simulink library "vmc"  (R2021b)
settings: Solver=VariableStepAuto  StartTime=0.0  StopTime=10.0  RelTol=1e-3
undefined symbols (not defined in the file or in its folder): AVMC_ACCDeltaTqIGain_X_kph, AVMC_ACCDeltaTqIGain_Y_mps2, AVMC_ACCDeltaTqPGain_X_kph, AVMC_ACCDeltaTqPGain_Y_kph, AVMC_ACCLongSteadyCtrl_X_kph, AVMC_AggressJerkPCT4AT_X_kph, AVMC_AggressJerkPCT_X_kph, AVMC_AggressLimitPCT4AT_X_kph, AVMC_AggressLimitPCT_X_kph, AVMC_CCLongSteadyCtrl_X_kph, AVMC_DISCDeltaTqIGain_X_kph, AVMC_DISCDeltaTqIGain_Y_mps2, AVMC_DISCDeltaTqPGain_X_kph, AVMC_DISCDeltaTqPGain_Y_kph, AVMC_DISCTrunAccJerk_X_s, AVMC_DISCTrunAccLimit_X_s, AVMC_ESCRegenOut_X_kph, AVMC_ESCRegenOut_Y_Deg, AVMC_ESCRegenOutEnSpd_X_Deg, AVMC_ISOAccLimit_X_mps, AVMC_ISODecLimit_X_mps, AVMC_ISOJerk_X_mps, AVMC_LatESCRegenOut_X_kph, AVMC_LatESCRegenOut_Y_Deg, AVMC_LongAccDeadZone_X_kph, AVMC_LongAccFiltTsforP2_X_Gps, AVMC_MCPresBaseTq_X_bar, AVMC_MSALongSteadyCtrl_X_kph, AVMC_MSAPedalOvrd2_X_kph, AVMC_MSAPedalOvrd_X_kph, AVMC_MSASpdBand_X_kph, AVMC_MSATqDownEndTq_X_kph, AVMC_MSATqDownTime_X_kph, AVMC_RDCDetectTime_X_kph, AVMC_RDCDetectTime_Y_pct, AVMC_RDCEnSlideRate_X_Deg, AVMC_RearWhlTqRatio_X_Nm, AVMC_RearWhlTqRatio_Y_gps, AVMC_RearWhlTqSlipGain_X_rat, AVMC_RearWhlTqSlipGain_Y_kph, AVMC_SoftJerkPCT_X_kph, AVMC_SoftLimitPCT_X_kph, AVMC_StESCYaw_X_kph, AVMC_StESCYaw_Y_Deg, AVMC_StESCYawCom_X_kph, AVMC_StESCYawCom_Y_Gps, AVMC_TMSpdBaseTq_X_rpm, AVMC_VehHoldBDecMap_X_kph, AVMC_VehHoldDecCtrlTime_X_kph, AVMC_VehHoldMCPPass_X_deg, C_TASK_10MS_S, C_TASK_5MS_S, DEG2RAD, Discrete, ENUM_ACCAVAIL_AVAILABLE, ENUM_ACCCTRLALLOW_ALLOW, ENUM_ADASACCSTA_ACTIVE, ENUM_ADASACCSTA_OVERRIDE, ENUM_ADASACCSTA_SHUTOFF, ENUM_ADASAEBREQ_NOREQUEST ... (+361)
libraries: hcu_lib x63, simulink x60, simulink_extras x3, ctrlSharedLib x3, $bdroot x2
(part 5 of 15)

== system vmc/VMC/VMC/SpeedCalculation ==
  VINP_MeterIndVehSpeed_kph : Inport
  VINP_Distanceunit_flg : Inport  Port=2
  VINP_VehSpeed_kph : Inport  Port=3
  function : TriggerPort  TriggerType=function-call  VariantControl=(inherit)
  Add8 : Sum
  Cast To Single1 : DataTypeConversion  OutDataTypeStr=uint8
  Cast To Single{2..3,6..7,10..12} (7 alike) : DataTypeConversion  OutDataTypeStr=single
  Cast To Single13 : DataTypeConversion  OutDataTypeStr=uint8
  Constant1 : Constant  Value=KVMC_MeterSpdRoundSW_flg
  Constant11 : Constant  Value=KPH2MPH
  Constant19 : Constant  Value=KPH2MPH
  Constant2 : Constant  Value=KVMC_MeterSpdRoundSW_flg
  Constant22 : Constant  Value=C_TASK_10MS_S
  Constant23 : Constant  Value=KVMC_MeterSpdBWFilter_raw32
  Constant4 : Constant  Value=ONE_INT
  Constant5 : Constant  Value=KVMC_MeterSpdRollAveLevel_enum
  Constant7 : Constant  Value=ZERO_FLOAT
  Divide : Product  Inputs=**
  Divide2 : Product  Inputs=**
  FirstOrderFilter6 : hcu_lib/Basic_Blocks/FirstOrderFilter
  RollingAverage : Stateflow chart  TreatAsAtomicUnit=on
  Round : Rounding
  Round1 : Rounding  Operator=round
  Round2 : Rounding
  Round3 : Rounding  Operator=round
  u2 > 0 (1) : Switch  Criteria=u2 > Threshold
  u2 > 0 (1)1 : Switch  Criteria=u2 > Threshold
  u2 > 0 (1)2 : Switch  Criteria=u2 > Threshold
  VVMC_MeterIndSpeed_raw32 : Outport
  VVMC_VehicleSpeed_mph : Outport  Port=2
  VVMC_VehicleSpeed_kph : Outport  Port=3
  VVMC_MeterIndSpeedForCalcu_kph : Outport  Port=4
  wires:
  u2 > 0 (1)/1 -> Cast To Single6/1
  VINP_Distanceunit_flg/1 -> [VINP_Distanceunit_flg]
  [VINP_Distanceunit_flg] -> u2 > 0 (1)/2
  FirstOrderFilter6/1 -> [VVMC_MeterSpdRollAve_kph]  "VVMC_MeterSpdRollAve_kph"
  [VVMC_MeterIndSpeed_raw32] -> VVMC_MeterIndSpeed_raw32/1
  Constant19/1 -> Divide/2
  u2 > 0 (1)2/1 -> [VVMC_MeterIndSpeedForCalcu_kph]  "VVMC_MeterIndSpeedForCalcu_kph"
  [VVMC_VehicleSpeed_kph] -> VVMC_VehicleSpeed_kph/1
  Cast To Single6/1 -> Round1/1, Round/1
  Constant11/1 -> Divide2/2
  Cast To Single2/1 -> Divide2/1
  [VVMC_MeterIndSpeedForCalcu_kph] -> VVMC_MeterIndSpeedForCalcu_kph/1
  u2 > 0 (1)1/1 -> [VVMC_MeterIndSpeed_raw32]  "VVMC_MeterIndSpeed_raw32"
  VINP_VehSpeed_kph/1 -> [VINP_VehSpeed_kph]
  Divide/1 -> u2 > 0 (1)/1
  [VVMC_MeterSpdRollAve_kph] -> Cast To Single7/1, u2 > 0 (1)/3, Round2/1, Round3/1  "VVMC_MeterSpdRollAve_kph"
  [VINP_VehSpeed_kph] -> Cast To Single10/1, Cast To Single2/1
  Cast To Single7/1 -> Divide/1
  VINP_MeterIndVehSpeed_kph/1 -> [VINP_MeterIndVehSpeed_kph]
  Divide2/1 -> [VVMC_VehicleSpeed_mph]  "VVMC_VehicleSpeed_mph"
  Cast To Single10/1 -> [VVMC_VehicleSpeed_kph]  "VVMC_VehicleSpeed_kph"
  [VVMC_VehicleSpeed_mph] -> VVMC_VehicleSpeed_mph/1
  Constant22/1 -> Add8/1, FirstOrderFilter6/2
  Add8/1 -> FirstOrderFilter6/3
  Constant23/1 -> Add8/2
  Cast To Single3/1 -> FirstOrderFilter6/1
  Constant1/1 -> u2 > 0 (1)1/2
  Round/1 -> u2 > 0 (1)1/3
  Round1/1 -> u2 > 0 (1)1/1
  Round2/1 -> u2 > 0 (1)2/3
  Constant2/1 -> u2 > 0 (1)2/2
  Round3/1 -> u2 > 0 (1)2/1
  RollingAverage/1(VVMC_MeterSpdRollAve_kph) -> Cast To Single3/1
  Constant5/1 -> Cast To Single1/1
  [VINP_MeterIndVehSpeed_kph] -> Cast To Single12/1
  Constant4/1 -> Cast To Single13/1
  Constant7/1 -> Cast To Single11/1
  Cast To Single12/1 -> RollingAverage/4(VINP_MeterIndVehSpeed_kph)
  Cast To Single13/1 -> RollingAverage/3(ONE_INT)
  Cast To Single11/1 -> RollingAverage/2(ZERO_FLOAT)
  Cast To Single1/1 -> RollingAverage/1(KVMC_MeterSpdRollAveLevel_enum)

== system vmc/VMC/VMC/Triggered Subsystem ==
  In1 : Inport
  Trigger : TriggerPort  VariantControl=(inherit)
  Out1 : Outport
  wires:
  In1/1 -> Out1/1

== system vmc/VMC/VMC/Triggered Subsystem1 ==
  In1 : Inport
  Trigger : TriggerPort  VariantControl=(inherit)
  Out1 : Outport
  wires:
  In1/1 -> Out1/1

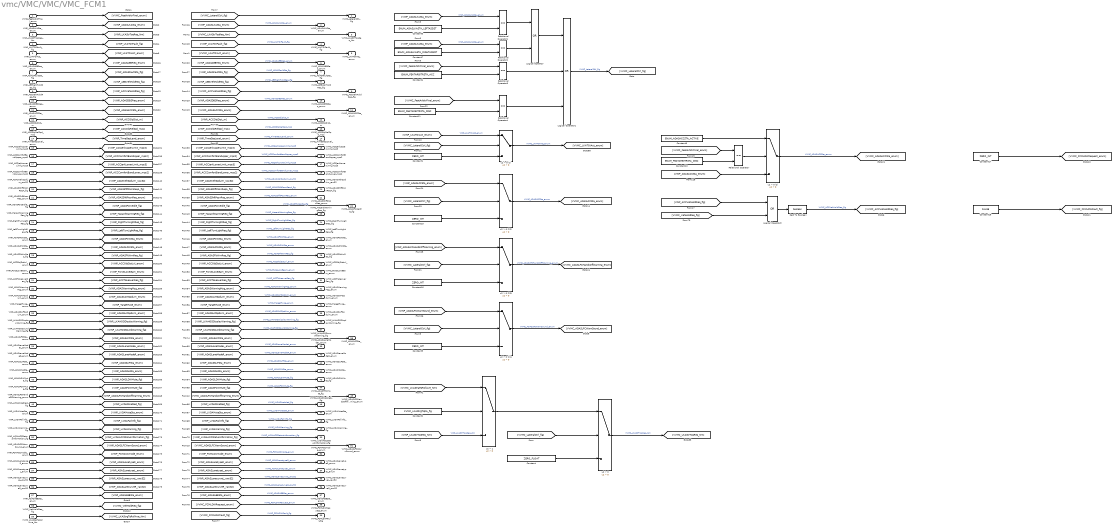
== system vmc/VMC/VMC/VMC_FCM1 ==
  VVMC_FeatArbitrFinal_enum : Inport
  VINP_ADASLKASta_enum : Inport  Port=2
  VINP_LKAStrToqReq_Nm : Inport  Port=3
  VINP_LKATOIFault_flg : Inport  Port=4
  VINP_LKATOIAct_enum : Inport  Port=5
  VINP_ADASAEBReq_enum : Inport  Port=6
  VINP_ADASFaultSta_flg : Inport  Port=7
  VINP_AEBVehHoldReq_flg : Inport  Port=8
  VINP_ACCVehHoldReq_flg : Inport  Port=9
  VINP_ADASDBSReq_enum : Inport  Port=10
  VINP_ADASACCSta_enum : Inport  Port=11
  VINP_ACCObjDist_m : Inport  Port=12
  VINP_ACCObjRelSpd_mps : Inport  Port=13
  VINP_TimeGapLevel_enum : Inport  Port=14
  VINP_ACCJerkUpperLimit_mps3 : Inport  Port=15
  VINP_ACCComfortBandUpper_mps2 : Inport  Port=16
  VINP_ACCJerkLowerLimit_mps3 : Inport  Port=17
  VINP_ACCComfortBandLower_mps2 : Inport  Port=18
  VINP_ADASVehSpdLim_raw32 : Inport  Port=19
  VINP_ADASShftPosnReqA_flg : Inport  Port=20
  VINP_ADASShftPosnReq_enum : Inport  Port=21
  VINP_ADASForceIdle_flg : Inport  Port=22
  VINP_HazardWarningReq_flg : Inport  Port=23
  VINP_RightTurnLightReq_flg : Inport  Port=24
  VINP_LeftTurnLightReq_flg : Inport  Port=25
  VINP_ADASFCWSta_enum : Inport  Port=26
  VINP_ADASLDWSta_enum : Inport  Port=27
  VINP_ADASFltWrnReq_flg : Inport  Port=28
  VINP_ACCObjDstLvl_enum : Inport  Port=29
  VINP_ForceLowBeam_enum : Inport  Port=30
  VINP_ACCTakeoverReq_flg : Inport  Port=31
  VINP_ADASWarningMsg_enum : Inport  Port=32
  VINP_ADASCAMSpdLim_enum : Inport  Port=33
  VINP_TargetType_enum : Inport  Port=34
  VINP_ADASSLIFSpdLim_enum : Inport  Port=35
  VINP_LKAHODDisplayWarning_flg : Inport  Port=36
  VINP_LKAHODSoundWarning_flg : Inport  Port=37
  VINP_ADASLFCSta_enum : Inport  Port=38
  VINP_ADASLaneModeL_enum : Inport  Port=39
  VINP_ADASLaneModeR_enum : Inport  Port=40
  VINP_ADASSLIFSta_enum : Inport  Port=41
  VINP_ADASISASta_enum : Inport  Port=42
  VINP_ADASLDWMute_flg : Inport  Port=43
  VINP_ADASFCWMute_flg : Inport  Port=44
  VINP_ADASLFCHandsOffWarning_enum : Inport  Port=45
  VINP_LVDADisabled_flg : Inport  Port=46
  VINP_LVDAMuteSta_enum : Inport  Port=47
  VINP_LVDAFailinfo_flg : Inport  Port=48
  VINP_LVDAWarning_flg : Inport  Port=49
  VINP_LVDAACCStatusInformation_flg : Inport  Port=50
  VINP_ADASLFCWarnSound_enum : Inport  Port=51
  VINP_FCMACCmode_enum : Inport  Port=52
  VINP_ADASLanetypeR_enum : Inport  Port=53
  VINP_ADASLanetypeL_enum : Inport  Port=54
  VINP_ADASLanecurveL_raw32 : Inport  Port=55
  VINP_ADASLanecurveR_raw32 : Inport  Port=56
  VINP_ADASAEBSta_enum : Inport  Port=57
  VVMC_VehHoldReq_flg : Inport  Port=58
  VVMC_LKAStrgTqRollAve_Nm : Inport  Port=59
  Cast To Boolean : DataTypeConversion  OutDataTypeStr=boolean
  Constant : Constant  Value=ZERO_FLOAT
  Constant{1,3,15..17} (5 alike) : Constant  Value=ZERO_INT
  Constant10 : Constant  Value=ENUM_FEATARBITRSTA_DISC
  Constant11 : Constant  Value=ENUM_FEATARBITRSTA_DISC
  Constant18 : Constant  Value=FALSE
  Constant2 : Constant  Value=KVMC_LKAStrgTqRA_flg
  Constant4 : Constant  Value=ENUM_FEATARBITRSTA_ACC
  Constant6 : Constant  Value=ENUM_ADASLKASTA_LEFTASSIST
  Constant7 : Constant  Value=ENUM_ADASLKASTA_RIGHTASSIST
  Constant9 : Constant  Value=ENUM_ADASACCSTA_ACTIVE
  Logical Operator : Logic  Operator=OR  AllPortsSameDT=off  OutDataTypeStr=boolean
  Logical Operator1 : Logic  Operator=OR  Inputs=3  AllPortsSameDT=off  OutDataTypeStr=boolean
  Logical Operator2 : Logic  Operator=OR  AllPortsSameDT=off  OutDataTypeStr=boolean
  Relational Operator{,1..4} (5 alike) : RelationalOperator  Operator===  OutDataTypeStr=boolean  RndMeth=Simplest
  u2 > 0 : Switch  Criteria=u2 > Threshold
  u2 > 0 (1) : Switch  Criteria=u2 > Threshold
  u2 > 0 (2){,2..4} (4 alike) : Switch  Criteria=u2 > Threshold
  u2 > 1 : Switch  Criteria=u2 > Threshold
  VVMC_LateralCtrl_flg : Outport
  VVMC_ADASLKASta_enum : Outport  Port=2
  VVMC_LKAStrToqReq_Nm : Outport  Port=3
  VVMC_LKATOIFault_flg : Outport  Port=4
  VVMC_LKATOIAct_enum : Outport  Port=5
  VVMC_ADASAEBReq_enum : Outport  Port=6
  VVMC_ADASFaultSta_flg : Outport  Port=7
  VVMC_AEBVehHoldReq_flg : Outport  Port=8
  VVMC_ACCVehHoldReq_flg : Outport  Port=9
  VVMC_ADASDBSReq_enum : Outport  Port=10
  VVMC_ADASACCSta_enum : Outport  Port=11
  VVMC_ACCObjDist_m : Outport  Port=12
  VVMC_ACCObjRelSpd_mps : Outport  Port=13
  VVMC_TimeGapLevel_enum : Outport  Port=14
  VVMC_ACCJerkUpperLimit_mps3 : Outport  Port=15
  VVMC_ACCComfortBandUpper_mps2 : Outport  Port=16
  VVMC_ACCJerkLowerLimit_mps3 : Outport  Port=17
  VVMC_ACCComfortBandLower_mps2 : Outport  Port=18
  VVMC_ADASVehSpdLim_raw32 : Outport  Port=19
  VVMC_ADASShftPosnReqA_flg : Outport  Port=20
  VVMC_ADASShftPosnReq_enum : Outport  Port=21
  VVMC_ADASForceIdle_flg : Outport  Port=22
  VVMC_HazardWarningReq_flg : Outport  Port=23
  VVMC_RightTurnLightReq_flg : Outport  Port=24
  VVMC_LeftTurnLightReq_flg : Outport  Port=25
  VVMC_ADASFCWSta_enum : Outport  Port=26
  VVMC_ADASLDWSta_enum : Outport  Port=27
  VVMC_ADASFltWrnReq_flg : Outport  Port=28
  VVMC_ACCObjDstLvl_enum : Outport  Port=29
  VVMC_ForceLowBeam_enum : Outport  Port=30
  VVMC_ACCTakeoverReq_flg : Outport  Port=31
  VVMC_ADASWarningMsg_enum : Outport  Port=32
  VVMC_ADASCAMSpdLim_enum : Outport  Port=33
  VVMC_TargetType_enum : Outport  Port=34
  VVMC_ADASSLIFSpdLim_enum : Outport  Port=35
  VVMC_LKAHODDisplayWarning_flg : Outport  Port=36
  VVMC_LKAHODSoundWarning_flg : Outport  Port=37
  VVMC_ADASLFCSta_enum : Outport  Port=38
  VVMC_ADASLaneModeL_enum : Outport  Port=39
  VVMC_ADASLaneModeR_enum : Outport  Port=40
  VVMC_ADASSLIFSta_enum : Outport  Port=41
  VVMC_ADASISASta_enum : Outport  Port=42
  VVMC_ADASLDWMute_flg : Outport  Port=43
  VVMC_ADASFCWMute_flg : Outport  Port=44
  VVMC_ADASLFCHandsOffWarning_enum : Outport  Port=45
  VVMC_LVDADisabled_flg : Outport  Port=46
  VVMC_LVDAMuteSta_enum : Outport  Port=47
  VVMC_LVDAFailinfo_flg : Outport  Port=48
  VVMC_LVDAWarning_flg : Outport  Port=49
  VVMC_LVDAACCStatusInformation_flg : Outport  Port=50
  VVMC_ADASLFCWarnSound_enum : Outport  Port=51
  VVMC_FCMACCmode_enum : Outport  Port=52
  VVMC_ADASLanetypeR_enum : Outport  Port=53
  VVMC_ADASLanetypeL_enum : Outport  Port=54
  VVMC_ADASLanecurveL_raw32 : Outport  Port=55
  VVMC_ADASLanecurveR_raw32 : Outport  Port=56
  VVMC_ADASAEBSta_enum : Outport  Port=57
  VVMC_FCMLDWRequest_enum : Outport  Port=58
  VVMC_FCMLDWFault_flg : Outport  Port=59
  wires:
  [VVMC_LateralCtrl_flg] -> VVMC_LateralCtrl_flg/1
  u2 > 0 (1)/1 -> [VVMC_LKATOIAct_enum]  "VVMC_LKATOIAct_enum"
  Constant1/1 -> u2 > 0 (1)/3
  [VVMC_LateralCtrl_flg] -> u2 > 0 (1)/2
  u2 > 0/1 -> [VVMC_LKAStrToqReq_Nm]  "VVMC_LKAStrToqReq_Nm"
  Constant/1 -> u2 > 0/3
  [VVMC_LateralCtrl_flg] -> u2 > 0/2
  Logical Operator1/1 -> [VVMC_LateralCtrl_flg]  "VVMC_LateralCtrl_flg"
  Relational Operator3/1 -> Logical Operator1/2
  Logical Operator/1 -> Logical Operator1/1
  Relational Operator2/1 -> Logical Operator/2
  Relational Operator1/1 -> Logical Operator/1
  [VINP_ADASLKASta_enum] -> Relational Operator2/1  "VINP_ADASLKASta_enum"
  [VINP_ADASLKASta_enum] -> Relational Operator1/1  "VINP_ADASLKASta_enum"
  [VVMC_FeatArbitrFinal_enum] -> Relational Operator3/1
  Constant4/1 -> Relational Operator3/2
  Constant6/1 -> Relational Operator1/2
  Constant7/1 -> Relational Operator2/2
  u2 > 1/1 -> u2 > 0/1
  [VINP_LKATOIAct_enum] -> u2 > 0 (1)/1  "VINP_LKATOIAct_enum"
  VINP_LKATOIAct_enum/1 -> [VINP_LKATOIAct_enum]
  VINP_LKATOIFault_flg/1 -> [VINP_LKATOIFault_flg]
  VINP_LKAStrToqReq_Nm/1 -> [VINP_LKAStrToqReq_Nm]
  VINP_ADASLKASta_enum/1 -> [VINP_ADASLKASta_enum]
  VVMC_FeatArbitrFinal_enum/1 -> [VVMC_FeatArbitrFinal_enum]
  VINP_ADASFaultSta_flg/1 -> [VINP_ADASFaultSta_flg]
  VINP_ADASAEBReq_enum/1 -> [VINP_ADASAEBReq_enum]
  VINP_AEBVehHoldReq_flg/1 -> [VINP_AEBVehHoldReq_flg]
  VINP_ADASDBSReq_enum/1 -> [VINP_ADASDBSReq_enum]
  VINP_ACCVehHoldReq_flg/1 -> [VINP_ACCVehHoldReq_flg]
  [VINP_ADASACCSta_enum] -> u2 > 0 (2)/3
  u2 > 0 (2)/1 -> [VVMC_ADASACCSta_enum]  "VVMC_ADASACCSta_enum"
  [VVMC_FeatArbitrFinal_enum] -> Relational Operator/1
  VINP_ADASACCSta_enum/1 -> [VINP_ADASACCSta_enum]
  Constant9/1 -> u2 > 0 (2)/1
  Constant10/1 -> Relational Operator/2
  Relational Operator/1 -> u2 > 0 (2)/2
  VINP_ACCJerkUpperLimit_mps3/1 -> [VINP_ACCJerkUpperLimit_mps3]
  VINP_ForceLowBeam_enum/1 -> [VINP_ForceLowBeam_enum]
  VINP_ADASLFCSta_enum/1 -> [VINP_ADASLFCSta_enum]
  VINP_ADASLanecurveR_raw32/1 -> [VINP_ADASLanecurveR_raw32]
  VINP_ADASLDWSta_enum/1 -> [VINP_ADASLDWSta_enum]
  VINP_ADASLaneModeR_enum/1 -> [VINP_ADASLaneModeR_enum]
  VINP_ACCComfortBandLower_mps2/1 -> [VINP_ACCComfortBandLower_mps2]
  VINP_ADASLanecurveL_raw32/1 -> [VINP_ADASLanecurveL_raw32]
  VINP_TargetType_enum/1 -> [VINP_TargetType_enum]
  VINP_ACCJerkLowerLimit_mps3/1 -> [VINP_ACCJerkLowerLimit_mps3]
  VINP_ADASShftPosnReq_enum/1 -> [VINP_ADASShftPosnReq_enum]
  VINP_ADASSLIFSta_enum/1 -> [VINP_ADASSLIFSta_enum]
  VINP_ADASShftPosnReqA_flg/1 -> [VINP_ADASShftPosnReqA_flg]
  VINP_LVDAMuteSta_enum/1 -> [VINP_LVDAMuteSta_enum]
  VINP_ACCComfortBandUpper_mps2/1 -> [VINP_ACCComfortBandUpper_mps2]
  VINP_FCMACCmode_enum/1 -> [VINP_FCMACCmode_enum]
  VINP_ADASCAMSpdLim_enum/1 -> [VINP_ADASCAMSpdLim_enum]
  VINP_LVDADisabled_flg/1 -> [VINP_LVDADisabled_flg]
  VINP_LKAHODDisplayWarning_flg/1 -> [VINP_LKAHODDisplayWarning_flg]
  VINP_ADASLDWMute_flg/1 -> [VINP_ADASLDWMute_flg]
  VINP_ADASFCWSta_enum/1 -> [VINP_ADASFCWSta_enum]
  VINP_LKAHODSoundWarning_flg/1 -> [VINP_LKAHODSoundWarning_flg]
  VINP_LeftTurnLightReq_flg/1 -> [VINP_LeftTurnLightReq_flg]
  VINP_ADASWarningMsg_enum/1 -> [VINP_ADASWarningMsg_enum]
  VINP_ADASFCWMute_flg/1 -> [VINP_ADASFCWMute_flg]
  VINP_ADASLanetypeL_enum/1 -> [VINP_ADASLanetypeL_enum]
  VINP_ADASFltWrnReq_flg/1 -> [VINP_ADASFltWrnReq_flg]
  VINP_RightTurnLightReq_flg/1 -> [VINP_RightTurnLightReq_flg]
  VINP_ACCTakeoverReq_flg/1 -> [VINP_ACCTakeoverReq_flg]
  VINP_ADASLFCWarnSound_enum/1 -> [VINP_ADASLFCWarnSound_enum]
  VINP_ACCObjDstLvl_enum/1 -> [VINP_ACCObjDstLvl_enum]
  VINP_LVDAFailinfo_flg/1 -> [VINP_LVDAFailinfo_flg]
  VINP_HazardWarningReq_flg/1 -> [VINP_HazardWarningReq_flg]
  VINP_ADASSLIFSpdLim_enum/1 -> [VINP_ADASSLIFSpdLim_enum]
  VINP_LVDAWarning_flg/1 -> [VINP_LVDAWarning_flg]
  VINP_ADASLFCHandsOffWarning_enum/1 -> [VINP_ADASLFCHandsOffWarning_enum]
  VINP_ADASLaneModeL_enum/1 -> [VINP_ADASLaneModeL_enum]
  VINP_ADASLanetypeR_enum/1 -> [VINP_ADASLanetypeR_enum]
  VINP_LVDAACCStatusInformation_flg/1 -> [VINP_LVDAACCStatusInformation_flg]
  VINP_ADASVehSpdLim_raw32/1 -> [VINP_ADASVehSpdLim_raw32]
  VINP_ADASForceIdle_flg/1 -> [VINP_ADASForceIdle_flg]
  VINP_ADASISASta_enum/1 -> [VINP_ADASISASta_enum]
  VINP_ACCObjRelSpd_mps/1 -> [VINP_ACCObjRelSpd_mps]
  VINP_ACCObjDist_m/1 -> [VINP_ACCObjDist_m]
  VINP_TimeGapLevel_enum/1 -> [VINP_TimeGapLevel_enum]
  [VINP_ACCVehHoldReq_flg] -> Logical Operator2/1
  Cast To Boolean/1 -> [VVMC_ACCVehHoldReq_flg]  "VVMC_ACCVehHoldReq_flg"
  Constant15/1 -> u2 > 0 (2)2/3
  u2 > 0 (2)2/1 -> [VVMC_ADASLFCSta_enum]  "VVMC_ADASLFCSta_enum"
  [VINP_ADASLFCSta_enum] -> u2 > 0 (2)2/1
  [VVMC_LateralCtrl_flg] -> u2 > 0 (2)2/2
  [VVMC_LateralCtrl_flg] -> u2 > 0 (2)3/2
  [VINP_ADASLFCHandsOffWarning_enum] -> u2 > 0 (2)3/1
  u2 > 0 (2)3/1 -> [VVMC_ADASLFCHandsOffWarning_enum]  "VVMC_ADASLFCHandsOffWarning_enum"
  Constant16/1 -> u2 > 0 (2)3/3
  Constant3/1 -> u2 > 0 (2)4/3
  u2 > 0 (2)4/1 -> [VVMC_ADASLFCWarnSound_enum]  "VVMC_ADASLFCWarnSound_enum"
  [VINP_ADASLFCWarnSound_enum] -> u2 > 0 (2)4/1
  [VVMC_LateralCtrl_flg] -> u2 > 0 (2)4/2
  [VINP_ADASLKASta_enum] -> VVMC_ADASLKASta_enum/1  "VVMC_ADASLKASta_enum"
  [VVMC_LKAStrToqReq_Nm] -> VVMC_LKAStrToqReq_Nm/1
  [VINP_LKATOIFault_flg] -> VVMC_LKATOIFault_flg/1  "VVMC_LKATOIFault_flg"
  [VVMC_LKATOIAct_enum] -> VVMC_LKATOIAct_enum/1
  [VINP_ADASAEBReq_enum] -> VVMC_ADASAEBReq_enum/1  "VVMC_ADASAEBReq_enum"
  [VINP_ADASFaultSta_flg] -> VVMC_ADASFaultSta_flg/1  "VVMC_ADASFaultSta_flg"
  [VINP_AEBVehHoldReq_flg] -> VVMC_AEBVehHoldReq_flg/1  "VVMC_AEBVehHoldReq_flg"
  [VVMC_ACCVehHoldReq_flg] -> VVMC_ACCVehHoldReq_flg/1
  [VINP_ADASDBSReq_enum] -> VVMC_ADASDBSReq_enum/1  "VVMC_ADASDBSReq_enum"
  [VVMC_ADASACCSta_enum] -> VVMC_ADASACCSta_enum/1
  [VINP_ACCObjDist_m] -> VVMC_ACCObjDist_m/1  "VVMC_ACCObjDist_m"
  [VINP_ACCObjRelSpd_mps] -> VVMC_ACCObjRelSpd_mps/1  "VVMC_ACCObjRelSpd_mps"
  [VINP_TimeGapLevel_enum] -> VVMC_TimeGapLevel_enum/1  "VVMC_TimeGapLevel_enum"
  [VINP_ACCJerkUpperLimit_mps3] -> VVMC_ACCJerkUpperLimit_mps3/1  "VVMC_ACCJerkUpperLimit_mps3"
  [VINP_ACCComfortBandUpper_mps2] -> VVMC_ACCComfortBandUpper_mps2/1  "VVMC_ACCComfortBandUpper_mps2"
  [VINP_ACCJerkLowerLimit_mps3] -> VVMC_ACCJerkLowerLimit_mps3/1  "VVMC_ACCJerkLowerLimit_mps3"
  [VINP_ACCComfortBandLower_mps2] -> VVMC_ACCComfortBandLower_mps2/1  "VVMC_ACCComfortBandLower_mps2"
  [VINP_ADASVehSpdLim_raw32] -> VVMC_ADASVehSpdLim_raw32/1  "VVMC_ADASVehSpdLim_raw32"
  [VINP_ADASShftPosnReqA_flg] -> VVMC_ADASShftPosnReqA_flg/1  "VVMC_ADASShftPosnReqA_flg"
  [VINP_ADASShftPosnReq_enum] -> VVMC_ADASShftPosnReq_enum/1  "VVMC_ADASShftPosnReq_enum"
  [VINP_ADASForceIdle_flg] -> VVMC_ADASForceIdle_flg/1  "VVMC_ADASForceIdle_flg"
  [VINP_HazardWarningReq_flg] -> VVMC_HazardWarningReq_flg/1  "VVMC_HazardWarningReq_flg"
  [VINP_RightTurnLightReq_flg] -> VVMC_RightTurnLightReq_flg/1  "VVMC_RightTurnLightReq_flg"
  [VINP_LeftTurnLightReq_flg] -> VVMC_LeftTurnLightReq_flg/1  "VVMC_LeftTurnLightReq_flg"
  [VINP_ADASFCWSta_enum] -> VVMC_ADASFCWSta_enum/1  "VVMC_ADASFCWSta_enum"
  [VINP_ADASLDWSta_enum] -> VVMC_ADASLDWSta_enum/1  "VVMC_ADASLDWSta_enum"
  [VINP_ADASFltWrnReq_flg] -> VVMC_ADASFltWrnReq_flg/1  "VVMC_ADASFltWrnReq_flg"
  [VINP_ACCObjDstLvl_enum] -> VVMC_ACCObjDstLvl_enum/1  "VVMC_ACCObjDstLvl_enum"
  [VINP_ForceLowBeam_enum] -> VVMC_ForceLowBeam_enum/1  "VVMC_ForceLowBeam_enum"
  [VINP_ACCTakeoverReq_flg] -> VVMC_ACCTakeoverReq_flg/1  "VVMC_ACCTakeoverReq_flg"
  [VINP_ADASWarningMsg_enum] -> VVMC_ADASWarningMsg_enum/1  "VVMC_ADASWarningMsg_enum"
  [VINP_ADASCAMSpdLim_enum] -> VVMC_ADASCAMSpdLim_enum/1  "VVMC_ADASCAMSpdLim_enum"
  [VINP_TargetType_enum] -> VVMC_TargetType_enum/1  "VVMC_TargetType_enum"
  [VINP_ADASSLIFSpdLim_enum] -> VVMC_ADASSLIFSpdLim_enum/1  "VVMC_ADASSLIFSpdLim_enum"
  [VINP_LKAHODDisplayWarning_flg] -> VVMC_LKAHODDisplayWarning_flg/1  "VVMC_LKAHODDisplayWarning_flg"
  [VINP_LKAHODSoundWarning_flg] -> VVMC_LKAHODSoundWarning_flg/1  "VVMC_LKAHODSoundWarning_flg"
  [VVMC_ADASLFCSta_enum] -> VVMC_ADASLFCSta_enum/1
  [VINP_ADASLaneModeL_enum] -> VVMC_ADASLaneModeL_enum/1  "VVMC_ADASLaneModeL_enum"
  [VINP_ADASLaneModeR_enum] -> VVMC_ADASLaneModeR_enum/1  "VVMC_ADASLaneModeR_enum"
  [VINP_ADASSLIFSta_enum] -> VVMC_ADASSLIFSta_enum/1  "VVMC_ADASSLIFSta_enum"
  [VINP_ADASISASta_enum] -> VVMC_ADASISASta_enum/1  "VVMC_ADASISASta_enum"
  [VINP_ADASLDWMute_flg] -> VVMC_ADASLDWMute_flg/1  "VVMC_ADASLDWMute_flg"
  [VINP_ADASFCWMute_flg] -> VVMC_ADASFCWMute_flg/1  "VVMC_ADASFCWMute_flg"
  [VVMC_ADASLFCHandsOffWarning_enum] -> VVMC_ADASLFCHandsOffWarning_enum/1
  [VINP_LVDADisabled_flg] -> VVMC_LVDADisabled_flg/1  "VVMC_LVDADisabled_flg"
  [VINP_LVDAMuteSta_enum] -> VVMC_LVDAMuteSta_enum/1  "VVMC_LVDAMuteSta_enum"
  [VINP_LVDAFailinfo_flg] -> VVMC_LVDAFailinfo_flg/1  "VVMC_LVDAFailinfo_flg"
  [VINP_LVDAWarning_flg] -> VVMC_LVDAWarning_flg/1  "VVMC_LVDAWarning_flg"
  [VINP_LVDAACCStatusInformation_flg] -> VVMC_LVDAACCStatusInformation_flg/1  "VVMC_LVDAACCStatusInformation_flg"
  [VVMC_ADASLFCWarnSound_enum] -> VVMC_ADASLFCWarnSound_enum/1
  [VINP_FCMACCmode_enum] -> VVMC_FCMACCmode_enum/1  "VVMC_FCMACCmode_enum"
  [VINP_ADASLanetypeR_enum] -> VVMC_ADASLanetypeR_enum/1  "VVMC_ADASLanetypeR_enum"
  [VINP_ADASLanetypeL_enum] -> VVMC_ADASLanetypeL_enum/1  "VVMC_ADASLanetypeL_enum"
  [VINP_ADASLanecurveL_raw32] -> VVMC_ADASLanecurveL_raw32/1  "VVMC_ADASLanecurveL_raw32"
  [VINP_ADASLanecurveR_raw32] -> VVMC_ADASLanecurveR_raw32/1  "VVMC_ADASLanecurveR_raw32"
  VINP_ADASAEBSta_enum/1 -> [VINP_ADASAEBSta_enum]
  [VINP_ADASAEBSta_enum] -> VVMC_ADASAEBSta_enum/1  "VVMC_ADASAEBSta_enum"
  Constant17/1 -> [VVMC_FCMLDWRequest_enum]
  Constant18/1 -> [VVMC_FCMLDWFault_flg]
  [VVMC_FCMLDWRequest_enum] -> VVMC_FCMLDWRequest_enum/1  "VVMC_FCMLDWRequest_enum"
  [VVMC_FCMLDWFault_flg] -> VVMC_FCMLDWFault_flg/1  "VVMC_FCMLDWFault_flg"
  VVMC_VehHoldReq_flg/1 -> [VVMC_VehHoldReq_flg]
  Logical Operator2/1 -> Cast To Boolean/1
  [VVMC_VehHoldReq_flg] -> Logical Operator2/2
  Constant11/1 -> Relational Operator4/2
  [VVMC_FeatArbitrFinal_enum] -> Relational Operator4/1
  Relational Operator4/1 -> Logical Operator1/3
  Constant2/1 -> u2 > 1/2
  [VINP_LKAStrToqReq_Nm] -> u2 > 1/3  "VINP_LKAStrToqReq_Nm"
  [VVMC_LKAStrgTqRollAve_Nm] -> u2 > 1/1
  VVMC_LKAStrgTqRollAve_Nm/1 -> [VVMC_LKAStrgTqRollAve_Nm]

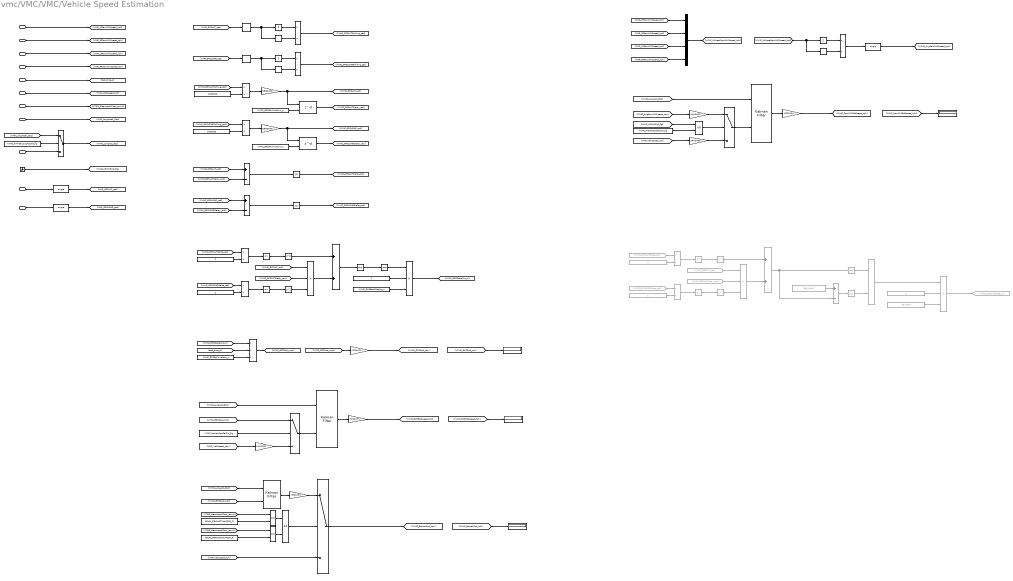
== system vmc/VMC/VMC/Vehicle Speed Estimation ==
  note: GPS
  note: RawWhl
  VINP_LFRawWhlSpeed_kph : Inport
  VINP_RFRawWhlSpeed_kph : Inport  Port=2
  VINP_LRRawWhlSpeed_kph : Inport  Port=3
  VINP_RRRawWhlSpeed_kph : Inport  Port=4
  VINP_VehSpeed_kph : Inport  Port=5
  VINP_LongAccel_Gps : Inport  Port=6
  VINP_GPSLAT_sec : Inport  Port=7
  VINP_GPSLONG_sec : Inport  Port=8
  VVMC_LongAcc_Gps : Inport  Port=9
  task_time_s : Inport  Port=10
  VTQD_GearActualPosn_enum : Inport  Port=11
  Abs : Abs
  Abs1 : Abs
  Asin : Trigonometry  Operator=asin
  Atan1 : Trigonometry  Commented=on  Operator=atan2
  Constant : Constant  Value=1000000  OutDataTypeStr=single
  Constant1 : Constant  Value=1000000  OutDataTypeStr=single
  Constant10 : Constant  Value=KVMC_PreVehSpdCalSW_flg
  Constant11 : Constant  Commented=on  Value=ONE_FLOAT  OutDataTypeStr=single
  Constant12 : Constant  Commented=on  Value=2  OutDataTypeStr=single
  Constant13 : Constant  Commented=on  Value=6371004  OutDataTypeStr=single
  Constant14 : Constant  Value=KVMC_PreVehSpdCalSW_flg
  Constant15 : Constant  Value=KVMC_GPSRollAveNum_c  OutDataTypeStr=single
  Constant16 : Constant  Value=KVMC_GPSRollAveNum_c  OutDataTypeStr=single
  Constant2 : Constant  Commented=on  Value=2  OutDataTypeStr=single
  Constant3 : Constant  Value=KVMC_4WheelLongAccSW_flg
  Constant4 : Constant  Commented=on  Value=2  OutDataTypeStr=single
  Constant46 : Constant  Value=ENUM_GEARACTUALPOSN_D
  Constant47 : Constant  Value=ENUM_GEARACTUALPOSN_R
  Constant5 : Constant  Value=2  OutDataTypeStr=single
  Constant6 : Constant  Value=2  OutDataTypeStr=single
  Constant7 : Constant  Value=KVMC_GPSRollAveNum_c  OutDataTypeStr=single
  Constant8 : Constant  Value=2  OutDataTypeStr=single
  Constant9 : Constant  Value=KVMC_GPSEarthRadius_c  OutDataTypeStr=single
  Data Type Conversion : DataTypeConversion  OutDataTypeStr=single
  Data Type Conversion1 : DataTypeConversion  OutDataTypeStr=single
  Data Type Conversion2 : DataTypeConversion  OutDataTypeStr=single
  Delay : Delay  DelayLengthSource=Input port  DelayLength=50  DelayLengthUpperLimit=5000
      settings: InputPortMap=u0,p1
  Delay1 : Delay  DelayLengthSource=Input port  DelayLength=50  DelayLengthUpperLimit=5000
      settings: InputPortMap=u0,p1
  Display{,1..3} (4 alike) : Display
  Divide{,1..3} (4 alike) : Product  Inputs=*/
  Divide10 : Product  Commented=on  Inputs=***
  Divide4 : Product  Inputs=***
  Divide5 : Product  Inputs=***
  Divide6 : Product  Inputs=*//
  Divide7 : Product  Commented=on  Inputs=*/
  Divide8 : Product  Commented=on  Inputs=*/
  Divide9 : Product  Commented=on  Inputs=***
  Equal : RelationalOperator  Operator===  OutDataTypeStr=boolean  RndMeth=Simplest
  Equal1 : RelationalOperator  Operator===  OutDataTypeStr=boolean  RndMeth=Simplest
  From13 : From  Commented=on  GotoTag=VVMC_GPSLATDelay_rad
  From15 : From  Commented=on  GotoTag=VVMC_GPSLATDelta_rad
  From32 : From  Commented=on  GotoTag=VVMC_GPSLONGDelta_rad
  From8 : From  Commented=on  GotoTag=VVMC_GPSLAT_rad
  Gain : Gain  Gain=DEG2RAD  OutDataTypeStr=single
  Gain1 : Gain  Gain=DEG2RAD  OutDataTypeStr=single
  Gain{2..4,6} (4 alike) : Gain  Gain=MPS2KPH  OutDataTypeStr=single
  Gain5 : Gain  Gain=KPH2MPS  OutDataTypeStr=single
  Gain7 : Gain  Gain=KPH2MPS  OutDataTypeStr=single
  Gain8 : Gain  Gain=KPH2MPS  OutDataTypeStr=single
  Goto25 : Goto  Commented=on  GotoTag=VVMC_GPSDisDelta_m
  Ground : Ground
  Kalman Filter1 : ctrlSharedLib/Kalman Filter  TimeDomain=Discrete-Time  UseCurrentEstimator=on  ModelSource=Individual A, B, C, D matrices  ModelSourceVariable=ss(0.95,1,1,0,1)  A=1  B=C_TASK_5MS_S  C=1  D=0  NumberOfStates=1  NumberOfInputs=1  NumberOfOutputs=1  InitialEstimateSource=Dialog  X0=0  P0=10  UseK=off  UseGH=off  NumberOfProcessNoiseInputs=1  G=1  TimeInvariantG=on  H=0  TimeInvariantH=on  Q=0.01  TimeInvariantQ=on  R=0.05  TimeInvariantR=on  N=0  TimeInvariantN=on  AddInputPort=on  AddEnablePort=off  OutputEstimatedY=off  OutputP=off  Ts=-1
  Kalman Filter2 : ctrlSharedLib/Kalman Filter  TimeDomain=Discrete-Time  UseCurrentEstimator=on  ModelSource=Individual A, B, C, D matrices  ModelSourceVariable=ss(0.95,1,1,0,1)  A=1  B=C_TASK_5MS_S  C=1  D=0  NumberOfStates=1  NumberOfInputs=1  NumberOfOutputs=1  InitialEstimateSource=Dialog  X0=0  P0=10  UseK=off  UseGH=off  NumberOfProcessNoiseInputs=1  G=1  TimeInvariantG=on  H=0  TimeInvariantH=on  Q=0.03  TimeInvariantQ=on  R=0.01  TimeInvariantR=on  N=0  TimeInvariantN=on  AddInputPort=on  AddEnablePort=off  OutputEstimatedY=off  OutputP=off  Ts=-1
  Kalman Filter3 : ctrlSharedLib/Kalman Filter  TimeDomain=Discrete-Time  UseCurrentEstimator=on  ModelSource=Individual A, B, C, D matrices  ModelSourceVariable=ss(0.95,1,1,0,1)  A=1  B=C_TASK_5MS_S  C=1  D=0  NumberOfStates=1  NumberOfInputs=1  NumberOfOutputs=1  InitialEstimateSource=Dialog  X0=0  P0=10  UseK=off  UseGH=off  NumberOfProcessNoiseInputs=1  G=1  TimeInvariantG=on  H=0  TimeInvariantH=on  Q=0.03  TimeInvariantQ=on  R=0.01  TimeInvariantR=on  N=0  TimeInvariantN=on  AddInputPort=on  AddEnablePort=off  OutputEstimatedY=off  OutputP=off  Ts=-1
  Minus : Sum  Inputs=+-
  Minus1 : Sum  Inputs=+-
  Minus2 : Sum
  Minus4 : Sum  Commented=on
  Minus5 : Sum  Commented=on  Inputs=+-
  Mux : Mux
  OR : Logic  Operator=OR  AllPortsSameDT=off  OutDataTypeStr=boolean
  OR1 : Logic  Operator=OR  AllPortsSameDT=off  OutDataTypeStr=boolean
  Product : Product  Inputs=*/
  Product2 : Product  Inputs=*/
  Product3 : Product  Inputs=*/
  Sin : Trigonometry
  Sin1 : Trigonometry
  Sin2 : Trigonometry  Commented=on
  Sin3 : Trigonometry  Commented=on
  Sqrt : Sqrt  SaturateOnIntegerOverflow=on
  Sqrt2 : Sqrt  Commented=on  SaturateOnIntegerOverflow=on
  Sqrt3 : Sqrt  Commented=on  SaturateOnIntegerOverflow=on
  Square : Math  Operator=square  SaturateOnIntegerOverflow=on
  Square1 : Math  Operator=square  SaturateOnIntegerOverflow=on
  Square2 : Math  Commented=on  Operator=square  SaturateOnIntegerOverflow=on
  Square3 : Math  Commented=on  Operator=square  SaturateOnIntegerOverflow=on
  Sum of Elements : Sum  Inputs=+
  Sum of Elements2 : Sum  Inputs=+
  Sum of Elements3 : Sum  Inputs=+
  Switch{,1..2,10} (4 alike) : Switch  Criteria=u2 > Threshold
  Tapped Delay1 : simulink/Discrete/Tapped Delay  vinit=0.0  samptime=-1  NumDelays=50  DelayOrder=Newest  includeCurrent=on
  Tapped Delay3 : simulink/Discrete/Tapped Delay  vinit=0.0  samptime=-1  NumDelays=50  DelayOrder=Newest  includeCurrent=on
  Width : Width
  Width2 : Width
  Width3 : Width
  wires:
  task_time_s/1 -> [task_time_s]
  VINP_RRRawWhlSpeed_kph/1 -> [VINP_RRRawWhlSpeed_kph]
  VINP_RFRawWhlSpeed_kph/1 -> [VINP_RFRawWhlSpeed_kph]
  VINP_VehSpeed_kph/1 -> [VINP_VehSpeed_kph]
  VINP_LRRawWhlSpeed_kph/1 -> [VINP_LRRawWhlSpeed_kph]
  VINP_LFRawWhlSpeed_kph/1 -> [VINP_LFRawWhlSpeed_kph]
  VTQD_GearActualPosn_enum/1 -> [VTQD_GearActualPosn_enum]
  VINP_LongAccel_Gps/1 -> [VINP_LongAccel_Gps]
  [VTQD_GearActualPosn_enum] -> Equal1/1
  Constant47/1 -> Equal1/2
  Constant46/1 -> Equal/2
  Equal/1 -> OR/1
  [VINP_VehSpeed_kph] -> Switch10/3
  Switch10/1 -> [VVMC_EstVehSpd_kph]  "VVMC_EstVehSpd_kph"
  OR/1 -> Switch10/2
  Equal1/1 -> OR/2
  [VTQD_GearActualPosn_enum] -> Equal/1
  [VINP_LongAccel_Gps] -> Switch/1
  VVMC_LongAcc_Gps/1 -> Switch/3
  Switch/1 -> [VVMC_LongAcc_Gps]  "VVMC_LongAcc_Gps"
  Constant3/1 -> Switch/2
  [VVMC_LongAcc_Gps] -> Kalman Filter1/1
  [VINP_LFRawWhlSpeed_kph] -> Mux/1
  [VINP_RRRawWhlSpeed_kph] -> Mux/4
  [VINP_LRRawWhlSpeed_kph] -> Mux/3
  [VINP_RFRawWhlSpeed_kph] -> Mux/2
  Mux/1 -> [VVMC_4WheelRawWhlSpeed_kph]
  Width/1 -> Product/2
  Sum of Elements/1 -> Product/1
  [VVMC_4WheelRawWhlSpeed_kph] -> Width/1, Sum of Elements/1
  [VVMC_GPSSpd_mps] -> Kalman Filter1/2
  Kalman Filter3/1 -> Gain4/1
  [VVMC_LongAcc_Gps] -> Kalman Filter3/1
  Ground/1 -> [VVMC_LFWhlSkid_flg]
  Product/1 -> Data Type Conversion/1
  Data Type Conversion/1 -> [VVMC_AvgRawWhlSpeed_kph]  "VVMC_AvgRawWhlSpeed_kph"
  [VVMC_EstVehSpd_kph] -> Display/1
  [VVMC_GPSLATRollAvg_sec] -> Divide/1
  Constant/1 -> Divide/2
  Constant1/1 -> Divide1/2
  [VVMC_GPSLONGRollAvg_sec] -> Divide1/1
  Delay/1 -> [VVMC_GPSLATDelay_rad]
  [VVMC_GPSLAT_rad] -> Minus/1
  Minus/1 -> Abs/1
  [VVMC_GPSLATDelay_rad] -> Minus/2
  Minus1/1 -> Abs1/1
  [VVMC_GPSLONG_rad] -> Minus1/1
  [VVMC_GPSLONGDelay_rad] -> Minus1/2
  Abs/1 -> [VVMC_GPSLATDelta_rad]
  Abs1/1 -> [VVMC_GPSLONGDelta_rad]
  [VVMC_GPSLATDelta_rad] -> Divide2/1
  Constant5/1 -> Divide2/2
  Divide2/1 -> Sin/1
  Sin/1 -> Square/1
  Constant6/1 -> Divide3/2
  [VVMC_GPSLONGDelta_rad] -> Divide3/1
  Divide3/1 -> Sin1/1
  Sin1/1 -> Square1/1
  Divide4/1 -> Minus2/2
  Square/1 -> Minus2/1
  [VVMC_GPSLATDelay_rad] -> Divide4/2
  [VVMC_GPSLAT_rad] -> Divide4/1
  Square1/1 -> Divide4/3
  Minus2/1 -> Sqrt/1
  Sqrt/1 -> Asin/1
  Asin/1 -> Divide5/1
  Constant8/1 -> Divide5/2
  Constant9/1 -> Divide5/3
  Divide5/1 -> [VVMC_GPSDeltaDis_m]
  Divide/1 -> Gain/1
  Gain/1 -> Delay/1, [VVMC_GPSLAT_rad]
  Divide1/1 -> Gain1/1
  [VINP_GPSLAT_sec] -> Tapped Delay1/1
  Width2/1 -> Product2/2
  Sum of Elements2/1 -> Product2/1
  Tapped Delay1/1 -> Sum of Elements2/1, Width2/1
  Product2/1 -> [VVMC_GPSLATRollAvg_sec]
  Product3/1 -> [VVMC_GPSLONGRollAvg_sec]
  Tapped Delay3/1 -> Width3/1, Sum of Elements3/1
  Sum of Elements3/1 -> Product3/1
  Width3/1 -> Product3/2
  [VINP_GPSLONG_sec] -> Tapped Delay3/1
  Kalman Filter1/1 -> Gain2/1
  Gain2/1 -> Switch10/1
  [VVMC_GPSSpd_mps] -> Gain3/1
  Gain3/1 -> [VVMC_GPSSpd_kph]  "VVMC_GPSSpd_kph"
  [VVMC_GPSSpd_kph] -> Display2/1
  Constant10/1 -> Switch2/2
  Switch2/1 -> Kalman Filter3/2
  [VVMC_GPSEstSpeed_kph] -> Display3/1
  Gain4/1 -> [VVMC_GPSEstSpeed_kph]  "VVMC_GPSEstSpeed_kph"
  Gain5/1 -> Switch2/3
  [VINP_VehSpeed_kph] -> Gain5/1
  [VVMC_GPSSpd_mps] -> Switch2/1
  Divide10/1 -> Goto25/1
  Constant13/1 -> Divide10/3
  Constant12/1 -> Divide10/2
  Atan1/1 -> Divide10/1
  Sqrt2/1 -> Atan1/1
  Sqrt3/1 -> Atan1/2
  Minus5/1 -> Sqrt3/1
  Constant11/1 -> Minus5/1
  Minus4/1 -> Sqrt2/1, Minus5/2
  Square3/1 -> Divide9/3
  From8/1 -> Divide9/1
  From13/1 -> Divide9/2
  Square2/1 -> Minus4/1
  Divide9/1 -> Minus4/2
  Sin3/1 -> Square3/1
  Divide8/1 -> Sin3/1
  From32/1 -> Divide8/1
  Constant4/1 -> Divide8/2
  Sin2/1 -> Square2/1
  Divide7/1 -> Sin2/1
  Constant2/1 -> Divide7/2
  From15/1 -> Divide7/1
  Constant7/1 -> Divide6/3
  [task_time_s] -> Divide6/2
  Divide6/1 -> [VVMC_GPSSpd_mps]
  [VVMC_GPSDeltaDis_m] -> Divide6/1
  Delay1/1 -> [VVMC_GPSLONGDelay_rad]
  [VINP_VehSpeed_kph] -> Gain7/1
  Gain7/1 -> Switch1/3
  Gain6/1 -> [VVMC_RawWhlEstSpeed_kph]  "VVMC_RawWhlEstSpeed_kph"
  [VVMC_RawWhlEstSpeed_kph] -> Display1/1
  Switch1/1 -> Kalman Filter2/2
  Constant14/1 -> OR1/2
  OR1/1 -> Switch1/2
  [VVMC_LFWhlSkid_flg] -> OR1/1
  [VVMC_LongAcc_Gps] -> Kalman Filter2/1
  Kalman Filter2/1 -> Gain6/1
  [VVMC_AvgRawWhlSpeed_kph] -> Gain8/1
  Gain8/1 -> Switch1/1
  VINP_GPSLAT_sec/1 -> Data Type Conversion1/1
  VINP_GPSLONG_sec/1 -> Data Type Conversion2/1
  Data Type Conversion1/1 -> [VINP_GPSLAT_sec]
  Data Type Conversion2/1 -> [VINP_GPSLONG_sec]
  Constant15/1 -> Delay/2
  Constant16/1 -> Delay1/2
  Gain1/1 -> Delay1/1, [VVMC_GPSLONG_rad]

== system vmc/VMC/VMC/ACC_Function/ACC Control Allow Judgement ==
  task_time_s : Inport
  VTQD_ExternalTqAllow_flag : Inport  Port=2
  VTQD_ExtDoorAllow_flg : Inport  Port=3
  AND : Logic  AllPortsSameDT=off  OutDataTypeStr=boolean
  Constant : Constant  Value=KVMC_ExternalTqAllowTime_s
  Constant3 : Constant  Value=TRUE
  Constant4 : Constant  Value=FALSE
  NOT : Logic  Operator=NOT  AllPortsSameDT=off  OutDataTypeStr=boolean
  Relational Operator : RelationalOperator  OutDataTypeStr=boolean  RndMeth=Simplest
  Timer : hcu_lib/Basic_Blocks/Timer
  u2>0 : Switch  Criteria=u2 > Threshold
  VVMC_ACCCtrlAllow_flg : Outport
  wires:
  task_time_s/1 -> [task_time_s]
  Constant/1 -> Relational Operator/2, Timer/4
  VTQD_ExternalTqAllow_flag/1 -> [VTQD_ExternalTqAllow_flag]
  NOT/1 -> Timer/2
  u2>0/1 -> [VVMC_ACCCtrlAllow_flg]  "VVMC_ACCCtrlAllow_flg"
  AND/1 -> NOT/1, Timer/1
  Constant4/1 -> u2>0/3
  Constant3/1 -> u2>0/1
  Timer/1 -> Relational Operator/1
  Relational Operator/1 -> u2>0/2
  [task_time_s] -> Timer/3
  [VVMC_ACCCtrlAllow_flg] -> VVMC_ACCCtrlAllow_flg/1
  [VTQD_ExtDoorAllow_flg] -> AND/2
  [VTQD_ExternalTqAllow_flag] -> AND/1
  VTQD_ExtDoorAllow_flg/1 -> [VTQD_ExtDoorAllow_flg]
